simulink model "cmult_core"  (R2013a)
settings: Solver=ode45  StartTime=0.0  StopTime=10.0  RelTol=1e-3
libraries: xbsIndex_r4 x2035, casper_library_misc x116, casper_library_multipliers x36
(part 8 of 23)

== system cmult_core/vaccs/cplx_vacc13 ==
  new_acc : Inport
  din : Inport  Port=2
  c_to_ri : casper_library_misc/c_to_ri  n_bits=17  bin_pt=0
      settings: AttributesFormatString=17_0 r/i
  ri_to_c : casper_library_misc/ri_to_c
  simple_bram_vacc36 : Subsystem  AncestorBlock=casper_library_accumulators/simple_bram_vacc  mask(simple_bram_vacc){vec_len=vacc_len, arith_type=Signed, n_bits=32, bin_pt=0}
      mask prompts: vec_len "Vector length:"; arith_type "Output type:"; n_bits "Bit width (output):"; bin_pt "Binary point (output):"
      mask help: This simple vector accumulator is based on a shift register. It outputs its previous accumulated vector after a new_acc pulse is received.
      mask init:
      | simple_bram_vacc_init(gcb, ...
      |     'vec_len', vec_len, ...
      |     'arith_type', arith_type, ...
      |     'n_bits', n_bits, ...
      |     'bin_pt', bin_pt);
      mask TypeOptions arith_type: Signed | Unsigned
  simple_bram_vacc37 : Subsystem  AncestorBlock=casper_library_accumulators/simple_bram_vacc  mask(simple_bram_vacc){vec_len=vacc_len, arith_type=Signed, n_bits=32, bin_pt=0}
      mask prompts: vec_len "Vector length:"; arith_type "Output type:"; n_bits "Bit width (output):"; bin_pt "Binary point (output):"
      mask help: This simple vector accumulator is based on a shift register. It outputs its previous accumulated vector after a new_acc pulse is received.
      mask init:
      | simple_bram_vacc_init(gcb, ...
      |     'vec_len', vec_len, ...
      |     'arith_type', arith_type, ...
      |     'n_bits', n_bits, ...
      |     'bin_pt', bin_pt);
      mask TypeOptions arith_type: Signed | Unsigned
  dout : Outport
  vld : Outport  Port=2
  wires:
  din/1 -> c_to_ri/1
  simple_bram_vacc36/2(valid) -> vld/1
  simple_bram_vacc37/1(dout) -> ri_to_c/2
  simple_bram_vacc36/1(dout) -> ri_to_c/1
  c_to_ri/2 -> simple_bram_vacc37/2(din)
  new_acc/1 -> simple_bram_vacc36/1(new_acc), simple_bram_vacc37/1(new_acc)
  c_to_ri/1 -> simple_bram_vacc36/2(din)
  simple_bram_vacc37/2(valid) -> ?
  ri_to_c/1 -> dout/1

== system cmult_core/vaccs/cplx_vacc14 ==
  new_acc : Inport
  din : Inport  Port=2
  c_to_ri : casper_library_misc/c_to_ri  n_bits=17  bin_pt=0
      settings: AttributesFormatString=17_0 r/i
  ri_to_c : casper_library_misc/ri_to_c
  simple_bram_vacc36 : Subsystem  AncestorBlock=casper_library_accumulators/simple_bram_vacc  mask(simple_bram_vacc){vec_len=vacc_len, arith_type=Signed, n_bits=32, bin_pt=0}
      mask prompts: vec_len "Vector length:"; arith_type "Output type:"; n_bits "Bit width (output):"; bin_pt "Binary point (output):"
      mask help: This simple vector accumulator is based on a shift register. It outputs its previous accumulated vector after a new_acc pulse is received.
      mask init:
      | simple_bram_vacc_init(gcb, ...
      |     'vec_len', vec_len, ...
      |     'arith_type', arith_type, ...
      |     'n_bits', n_bits, ...
      |     'bin_pt', bin_pt);
      mask TypeOptions arith_type: Signed | Unsigned
  simple_bram_vacc37 : Subsystem  AncestorBlock=casper_library_accumulators/simple_bram_vacc  mask(simple_bram_vacc){vec_len=vacc_len, arith_type=Signed, n_bits=32, bin_pt=0}
      mask prompts: vec_len "Vector length:"; arith_type "Output type:"; n_bits "Bit width (output):"; bin_pt "Binary point (output):"
      mask help: This simple vector accumulator is based on a shift register. It outputs its previous accumulated vector after a new_acc pulse is received.
      mask init:
      | simple_bram_vacc_init(gcb, ...
      |     'vec_len', vec_len, ...
      |     'arith_type', arith_type, ...
      |     'n_bits', n_bits, ...
      |     'bin_pt', bin_pt);
      mask TypeOptions arith_type: Signed | Unsigned
  dout : Outport
  vld : Outport  Port=2
  wires:
  ri_to_c/1 -> dout/1
  simple_bram_vacc37/2(valid) -> ?
  c_to_ri/1 -> simple_bram_vacc36/2(din)
  new_acc/1 -> simple_bram_vacc37/1(new_acc), simple_bram_vacc36/1(new_acc)
  c_to_ri/2 -> simple_bram_vacc37/2(din)
  simple_bram_vacc36/1(dout) -> ri_to_c/1
  simple_bram_vacc37/1(dout) -> ri_to_c/2
  simple_bram_vacc36/2(valid) -> vld/1
  din/1 -> c_to_ri/1

== system cmult_core/vaccs/cplx_vacc15 ==
  new_acc : Inport
  din : Inport  Port=2
  c_to_ri : casper_library_misc/c_to_ri  n_bits=17  bin_pt=0
      settings: AttributesFormatString=17_0 r/i
  ri_to_c : casper_library_misc/ri_to_c
  simple_bram_vacc36 : Subsystem  AncestorBlock=casper_library_accumulators/simple_bram_vacc  mask(simple_bram_vacc){vec_len=vacc_len, arith_type=Signed, n_bits=32, bin_pt=0}
      mask prompts: vec_len "Vector length:"; arith_type "Output type:"; n_bits "Bit width (output):"; bin_pt "Binary point (output):"
      mask help: This simple vector accumulator is based on a shift register. It outputs its previous accumulated vector after a new_acc pulse is received.
      mask init:
      | simple_bram_vacc_init(gcb, ...
      |     'vec_len', vec_len, ...
      |     'arith_type', arith_type, ...
      |     'n_bits', n_bits, ...
      |     'bin_pt', bin_pt);
      mask TypeOptions arith_type: Signed | Unsigned
  simple_bram_vacc37 : Subsystem  AncestorBlock=casper_library_accumulators/simple_bram_vacc  mask(simple_bram_vacc){vec_len=vacc_len, arith_type=Signed, n_bits=32, bin_pt=0}
      mask prompts: vec_len "Vector length:"; arith_type "Output type:"; n_bits "Bit width (output):"; bin_pt "Binary point (output):"
      mask help: This simple vector accumulator is based on a shift register. It outputs its previous accumulated vector after a new_acc pulse is received.
      mask init:
      | simple_bram_vacc_init(gcb, ...
      |     'vec_len', vec_len, ...
      |     'arith_type', arith_type, ...
      |     'n_bits', n_bits, ...
      |     'bin_pt', bin_pt);
      mask TypeOptions arith_type: Signed | Unsigned
  dout : Outport
  vld : Outport  Port=2
  wires:
  din/1 -> c_to_ri/1
  simple_bram_vacc36/2(valid) -> vld/1
  simple_bram_vacc37/1(dout) -> ri_to_c/2
  simple_bram_vacc36/1(dout) -> ri_to_c/1
  c_to_ri/2 -> simple_bram_vacc37/2(din)
  new_acc/1 -> simple_bram_vacc36/1(new_acc), simple_bram_vacc37/1(new_acc)
  c_to_ri/1 -> simple_bram_vacc36/2(din)
  simple_bram_vacc37/2(valid) -> ?
  ri_to_c/1 -> dout/1

== system cmult_core/vaccs/cplx_vacc16 ==
  new_acc : Inport
  din : Inport  Port=2
  c_to_ri : casper_library_misc/c_to_ri  n_bits=17  bin_pt=0
      settings: AttributesFormatString=17_0 r/i
  ri_to_c : casper_library_misc/ri_to_c
  simple_bram_vacc36 : Subsystem  AncestorBlock=casper_library_accumulators/simple_bram_vacc  mask(simple_bram_vacc){vec_len=vacc_len, arith_type=Signed, n_bits=32, bin_pt=0}
      mask prompts: vec_len "Vector length:"; arith_type "Output type:"; n_bits "Bit width (output):"; bin_pt "Binary point (output):"
      mask help: This simple vector accumulator is based on a shift register. It outputs its previous accumulated vector after a new_acc pulse is received.
      mask init:
      | simple_bram_vacc_init(gcb, ...
      |     'vec_len', vec_len, ...
      |     'arith_type', arith_type, ...
      |     'n_bits', n_bits, ...
      |     'bin_pt', bin_pt);
      mask TypeOptions arith_type: Signed | Unsigned
  simple_bram_vacc37 : Subsystem  AncestorBlock=casper_library_accumulators/simple_bram_vacc  mask(simple_bram_vacc){vec_len=vacc_len, arith_type=Signed, n_bits=32, bin_pt=0}
      mask prompts: vec_len "Vector length:"; arith_type "Output type:"; n_bits "Bit width (output):"; bin_pt "Binary point (output):"
      mask help: This simple vector accumulator is based on a shift register. It outputs its previous accumulated vector after a new_acc pulse is received.
      mask init:
      | simple_bram_vacc_init(gcb, ...
      |     'vec_len', vec_len, ...
      |     'arith_type', arith_type, ...
      |     'n_bits', n_bits, ...
      |     'bin_pt', bin_pt);
      mask TypeOptions arith_type: Signed | Unsigned
  dout : Outport
  vld : Outport  Port=2
  wires:
  din/1 -> c_to_ri/1
  simple_bram_vacc36/2(valid) -> vld/1
  simple_bram_vacc37/1(dout) -> ri_to_c/2
  simple_bram_vacc36/1(dout) -> ri_to_c/1
  c_to_ri/2 -> simple_bram_vacc37/2(din)
  new_acc/1 -> simple_bram_vacc36/1(new_acc), simple_bram_vacc37/1(new_acc)
  c_to_ri/1 -> simple_bram_vacc36/2(din)
  simple_bram_vacc37/2(valid) -> ?
  ri_to_c/1 -> dout/1

== system cmult_core/vaccs/cplx_vacc17 ==
  new_acc : Inport
  din : Inport  Port=2
  c_to_ri : casper_library_misc/c_to_ri  n_bits=17  bin_pt=0
      settings: AttributesFormatString=17_0 r/i
  ri_to_c : casper_library_misc/ri_to_c
  simple_bram_vacc36 : Subsystem  AncestorBlock=casper_library_accumulators/simple_bram_vacc  mask(simple_bram_vacc){vec_len=vacc_len, arith_type=Signed, n_bits=32, bin_pt=0}
      mask prompts: vec_len "Vector length:"; arith_type "Output type:"; n_bits "Bit width (output):"; bin_pt "Binary point (output):"
      mask help: This simple vector accumulator is based on a shift register. It outputs its previous accumulated vector after a new_acc pulse is received.
      mask init:
      | simple_bram_vacc_init(gcb, ...
      |     'vec_len', vec_len, ...
      |     'arith_type', arith_type, ...
      |     'n_bits', n_bits, ...
      |     'bin_pt', bin_pt);
      mask TypeOptions arith_type: Signed | Unsigned
  simple_bram_vacc37 : Subsystem  AncestorBlock=casper_library_accumulators/simple_bram_vacc  mask(simple_bram_vacc){vec_len=vacc_len, arith_type=Signed, n_bits=32, bin_pt=0}
      mask prompts: vec_len "Vector length:"; arith_type "Output type:"; n_bits "Bit width (output):"; bin_pt "Binary point (output):"
      mask help: This simple vector accumulator is based on a shift register. It outputs its previous accumulated vector after a new_acc pulse is received.
      mask init:
      | simple_bram_vacc_init(gcb, ...
      |     'vec_len', vec_len, ...
      |     'arith_type', arith_type, ...
      |     'n_bits', n_bits, ...
      |     'bin_pt', bin_pt);
      mask TypeOptions arith_type: Signed | Unsigned
  dout : Outport
  vld : Outport  Port=2
  wires:
  ri_to_c/1 -> dout/1
  simple_bram_vacc37/2(valid) -> ?
  c_to_ri/1 -> simple_bram_vacc36/2(din)
  new_acc/1 -> simple_bram_vacc37/1(new_acc), simple_bram_vacc36/1(new_acc)
  c_to_ri/2 -> simple_bram_vacc37/2(din)
  simple_bram_vacc36/1(dout) -> ri_to_c/1
  simple_bram_vacc37/1(dout) -> ri_to_c/2
  simple_bram_vacc36/2(valid) -> vld/1
  din/1 -> c_to_ri/1

== system cmult_core/vaccs/cplx_vacc18 ==
  new_acc : Inport
  din : Inport  Port=2
  c_to_ri : casper_library_misc/c_to_ri  n_bits=17  bin_pt=0
      settings: AttributesFormatString=17_0 r/i
  ri_to_c : casper_library_misc/ri_to_c
  simple_bram_vacc36 : Subsystem  AncestorBlock=casper_library_accumulators/simple_bram_vacc  mask(simple_bram_vacc){vec_len=vacc_len, arith_type=Signed, n_bits=32, bin_pt=0}
      mask prompts: vec_len "Vector length:"; arith_type "Output type:"; n_bits "Bit width (output):"; bin_pt "Binary point (output):"
      mask help: This simple vector accumulator is based on a shift register. It outputs its previous accumulated vector after a new_acc pulse is received.
      mask init:
      | simple_bram_vacc_init(gcb, ...
      |     'vec_len', vec_len, ...
      |     'arith_type', arith_type, ...
      |     'n_bits', n_bits, ...
      |     'bin_pt', bin_pt);
      mask TypeOptions arith_type: Signed | Unsigned
  simple_bram_vacc37 : Subsystem  AncestorBlock=casper_library_accumulators/simple_bram_vacc  mask(simple_bram_vacc){vec_len=vacc_len, arith_type=Signed, n_bits=32, bin_pt=0}
      mask prompts: vec_len "Vector length:"; arith_type "Output type:"; n_bits "Bit width (output):"; bin_pt "Binary point (output):"
      mask help: This simple vector accumulator is based on a shift register. It outputs its previous accumulated vector after a new_acc pulse is received.
      mask init:
      | simple_bram_vacc_init(gcb, ...
      |     'vec_len', vec_len, ...
      |     'arith_type', arith_type, ...
      |     'n_bits', n_bits, ...
      |     'bin_pt', bin_pt);
      mask TypeOptions arith_type: Signed | Unsigned
  dout : Outport
  vld : Outport  Port=2
  wires:
  din/1 -> c_to_ri/1
  simple_bram_vacc36/2(valid) -> vld/1
  simple_bram_vacc37/1(dout) -> ri_to_c/2
  simple_bram_vacc36/1(dout) -> ri_to_c/1
  c_to_ri/2 -> simple_bram_vacc37/2(din)
  new_acc/1 -> simple_bram_vacc36/1(new_acc), simple_bram_vacc37/1(new_acc)
  c_to_ri/1 -> simple_bram_vacc36/2(din)
  simple_bram_vacc37/2(valid) -> ?
  ri_to_c/1 -> dout/1

== system cmult_core/vaccs/cplx_vacc19 ==
  new_acc : Inport
  din : Inport  Port=2
  c_to_ri : casper_library_misc/c_to_ri  n_bits=17  bin_pt=0
      settings: AttributesFormatString=17_0 r/i
  ri_to_c : casper_library_misc/ri_to_c
  simple_bram_vacc36 : Subsystem  AncestorBlock=casper_library_accumulators/simple_bram_vacc  mask(simple_bram_vacc){vec_len=vacc_len, arith_type=Signed, n_bits=32, bin_pt=0}
      mask prompts: vec_len "Vector length:"; arith_type "Output type:"; n_bits "Bit width (output):"; bin_pt "Binary point (output):"
      mask help: This simple vector accumulator is based on a shift register. It outputs its previous accumulated vector after a new_acc pulse is received.
      mask init:
      | simple_bram_vacc_init(gcb, ...
      |     'vec_len', vec_len, ...
      |     'arith_type', arith_type, ...
      |     'n_bits', n_bits, ...
      |     'bin_pt', bin_pt);
      mask TypeOptions arith_type: Signed | Unsigned
  simple_bram_vacc37 : Subsystem  AncestorBlock=casper_library_accumulators/simple_bram_vacc  mask(simple_bram_vacc){vec_len=vacc_len, arith_type=Signed, n_bits=32, bin_pt=0}
      mask prompts: vec_len "Vector length:"; arith_type "Output type:"; n_bits "Bit width (output):"; bin_pt "Binary point (output):"
      mask help: This simple vector accumulator is based on a shift register. It outputs its previous accumulated vector after a new_acc pulse is received.
      mask init:
      | simple_bram_vacc_init(gcb, ...
      |     'vec_len', vec_len, ...
      |     'arith_type', arith_type, ...
      |     'n_bits', n_bits, ...
      |     'bin_pt', bin_pt);
      mask TypeOptions arith_type: Signed | Unsigned
  dout : Outport
  vld : Outport  Port=2
  wires:
  ri_to_c/1 -> dout/1
  simple_bram_vacc37/2(valid) -> ?
  c_to_ri/1 -> simple_bram_vacc36/2(din)
  new_acc/1 -> simple_bram_vacc37/1(new_acc), simple_bram_vacc36/1(new_acc)
  c_to_ri/2 -> simple_bram_vacc37/2(din)
  simple_bram_vacc36/1(dout) -> ri_to_c/1
  simple_bram_vacc37/1(dout) -> ri_to_c/2
  simple_bram_vacc36/2(valid) -> vld/1
  din/1 -> c_to_ri/1

== system cmult_core/vaccs/cplx_vacc2 ==
  new_acc : Inport
  din : Inport  Port=2
  c_to_ri : casper_library_misc/c_to_ri  n_bits=17  bin_pt=0
      settings: AttributesFormatString=17_0 r/i
  ri_to_c : casper_library_misc/ri_to_c
  simple_bram_vacc36 : Subsystem  AncestorBlock=casper_library_accumulators/simple_bram_vacc  mask(simple_bram_vacc){vec_len=vacc_len, arith_type=Signed, n_bits=32, bin_pt=0}
      mask prompts: vec_len "Vector length:"; arith_type "Output type:"; n_bits "Bit width (output):"; bin_pt "Binary point (output):"
      mask help: This simple vector accumulator is based on a shift register. It outputs its previous accumulated vector after a new_acc pulse is received.
      mask init:
      | simple_bram_vacc_init(gcb, ...
      |     'vec_len', vec_len, ...
      |     'arith_type', arith_type, ...
      |     'n_bits', n_bits, ...
      |     'bin_pt', bin_pt);
      mask TypeOptions arith_type: Signed | Unsigned
  simple_bram_vacc37 : Subsystem  AncestorBlock=casper_library_accumulators/simple_bram_vacc  mask(simple_bram_vacc){vec_len=vacc_len, arith_type=Signed, n_bits=32, bin_pt=0}
      mask prompts: vec_len "Vector length:"; arith_type "Output type:"; n_bits "Bit width (output):"; bin_pt "Binary point (output):"
      mask help: This simple vector accumulator is based on a shift register. It outputs its previous accumulated vector after a new_acc pulse is received.
      mask init:
      | simple_bram_vacc_init(gcb, ...
      |     'vec_len', vec_len, ...
      |     'arith_type', arith_type, ...
      |     'n_bits', n_bits, ...
      |     'bin_pt', bin_pt);
      mask TypeOptions arith_type: Signed | Unsigned
  dout : Outport
  vld : Outport  Port=2
  wires:
  din/1 -> c_to_ri/1
  simple_bram_vacc36/2(valid) -> vld/1
  simple_bram_vacc37/1(dout) -> ri_to_c/2
  simple_bram_vacc36/1(dout) -> ri_to_c/1
  c_to_ri/2 -> simple_bram_vacc37/2(din)
  new_acc/1 -> simple_bram_vacc36/1(new_acc), simple_bram_vacc37/1(new_acc)
  c_to_ri/1 -> simple_bram_vacc36/2(din)
  simple_bram_vacc37/2(valid) -> ?
  ri_to_c/1 -> dout/1

== system cmult_core/vaccs/cplx_vacc20 ==
  new_acc : Inport
  din : Inport  Port=2
  c_to_ri : casper_library_misc/c_to_ri  n_bits=17  bin_pt=0
      settings: AttributesFormatString=17_0 r/i
  ri_to_c : casper_library_misc/ri_to_c
  simple_bram_vacc36 : Subsystem  AncestorBlock=casper_library_accumulators/simple_bram_vacc  mask(simple_bram_vacc){vec_len=vacc_len, arith_type=Signed, n_bits=32, bin_pt=0}
      mask prompts: vec_len "Vector length:"; arith_type "Output type:"; n_bits "Bit width (output):"; bin_pt "Binary point (output):"
      mask help: This simple vector accumulator is based on a shift register. It outputs its previous accumulated vector after a new_acc pulse is received.
      mask init:
      | simple_bram_vacc_init(gcb, ...
      |     'vec_len', vec_len, ...
      |     'arith_type', arith_type, ...
      |     'n_bits', n_bits, ...
      |     'bin_pt', bin_pt);
      mask TypeOptions arith_type: Signed | Unsigned
  simple_bram_vacc37 : Subsystem  AncestorBlock=casper_library_accumulators/simple_bram_vacc  mask(simple_bram_vacc){vec_len=vacc_len, arith_type=Signed, n_bits=32, bin_pt=0}
      mask prompts: vec_len "Vector length:"; arith_type "Output type:"; n_bits "Bit width (output):"; bin_pt "Binary point (output):"
      mask help: This simple vector accumulator is based on a shift register. It outputs its previous accumulated vector after a new_acc pulse is received.
      mask init:
      | simple_bram_vacc_init(gcb, ...
      |     'vec_len', vec_len, ...
      |     'arith_type', arith_type, ...
      |     'n_bits', n_bits, ...
      |     'bin_pt', bin_pt);
      mask TypeOptions arith_type: Signed | Unsigned
  dout : Outport
  vld : Outport  Port=2
  wires:
  din/1 -> c_to_ri/1
  simple_bram_vacc36/2(valid) -> vld/1
  simple_bram_vacc37/1(dout) -> ri_to_c/2
  simple_bram_vacc36/1(dout) -> ri_to_c/1
  c_to_ri/2 -> simple_bram_vacc37/2(din)
  new_acc/1 -> simple_bram_vacc36/1(new_acc), simple_bram_vacc37/1(new_acc)
  c_to_ri/1 -> simple_bram_vacc36/2(din)
  simple_bram_vacc37/2(valid) -> ?
  ri_to_c/1 -> dout/1

== system cmult_core/vaccs/cplx_vacc21 ==
  new_acc : Inport
  din : Inport  Port=2
  c_to_ri : casper_library_misc/c_to_ri  n_bits=17  bin_pt=0
      settings: AttributesFormatString=17_0 r/i
  ri_to_c : casper_library_misc/ri_to_c
  simple_bram_vacc36 : Subsystem  AncestorBlock=casper_library_accumulators/simple_bram_vacc  mask(simple_bram_vacc){vec_len=vacc_len, arith_type=Signed, n_bits=32, bin_pt=0}
      mask prompts: vec_len "Vector length:"; arith_type "Output type:"; n_bits "Bit width (output):"; bin_pt "Binary point (output):"
      mask help: This simple vector accumulator is based on a shift register. It outputs its previous accumulated vector after a new_acc pulse is received.
      mask init:
      | simple_bram_vacc_init(gcb, ...
      |     'vec_len', vec_len, ...
      |     'arith_type', arith_type, ...
      |     'n_bits', n_bits, ...
      |     'bin_pt', bin_pt);
      mask TypeOptions arith_type: Signed | Unsigned
  simple_bram_vacc37 : Subsystem  AncestorBlock=casper_library_accumulators/simple_bram_vacc  mask(simple_bram_vacc){vec_len=vacc_len, arith_type=Signed, n_bits=32, bin_pt=0}
      mask prompts: vec_len "Vector length:"; arith_type "Output type:"; n_bits "Bit width (output):"; bin_pt "Binary point (output):"
      mask help: This simple vector accumulator is based on a shift register. It outputs its previous accumulated vector after a new_acc pulse is received.
      mask init:
      | simple_bram_vacc_init(gcb, ...
      |     'vec_len', vec_len, ...
      |     'arith_type', arith_type, ...
      |     'n_bits', n_bits, ...
      |     'bin_pt', bin_pt);
      mask TypeOptions arith_type: Signed | Unsigned
  dout : Outport
  vld : Outport  Port=2
  wires:
  ri_to_c/1 -> dout/1
  simple_bram_vacc37/2(valid) -> ?
  c_to_ri/1 -> simple_bram_vacc36/2(din)
  new_acc/1 -> simple_bram_vacc37/1(new_acc), simple_bram_vacc36/1(new_acc)
  c_to_ri/2 -> simple_bram_vacc37/2(din)
  simple_bram_vacc36/1(dout) -> ri_to_c/1
  simple_bram_vacc37/1(dout) -> ri_to_c/2
  simple_bram_vacc36/2(valid) -> vld/1
  din/1 -> c_to_ri/1

== system cmult_core/vaccs/cplx_vacc22 ==
  new_acc : Inport
  din : Inport  Port=2
  c_to_ri : casper_library_misc/c_to_ri  n_bits=17  bin_pt=0
      settings: AttributesFormatString=17_0 r/i
  ri_to_c : casper_library_misc/ri_to_c
  simple_bram_vacc36 : Subsystem  AncestorBlock=casper_library_accumulators/simple_bram_vacc  mask(simple_bram_vacc){vec_len=vacc_len, arith_type=Signed, n_bits=32, bin_pt=0}
      mask prompts: vec_len "Vector length:"; arith_type "Output type:"; n_bits "Bit width (output):"; bin_pt "Binary point (output):"
      mask help: This simple vector accumulator is based on a shift register. It outputs its previous accumulated vector after a new_acc pulse is received.
      mask init:
      | simple_bram_vacc_init(gcb, ...
      |     'vec_len', vec_len, ...
      |     'arith_type', arith_type, ...
      |     'n_bits', n_bits, ...
      |     'bin_pt', bin_pt);
      mask TypeOptions arith_type: Signed | Unsigned
  simple_bram_vacc37 : Subsystem  AncestorBlock=casper_library_accumulators/simple_bram_vacc  mask(simple_bram_vacc){vec_len=vacc_len, arith_type=Signed, n_bits=32, bin_pt=0}
      mask prompts: vec_len "Vector length:"; arith_type "Output type:"; n_bits "Bit width (output):"; bin_pt "Binary point (output):"
      mask help: This simple vector accumulator is based on a shift register. It outputs its previous accumulated vector after a new_acc pulse is received.
      mask init:
      | simple_bram_vacc_init(gcb, ...
      |     'vec_len', vec_len, ...
      |     'arith_type', arith_type, ...
      |     'n_bits', n_bits, ...
      |     'bin_pt', bin_pt);
      mask TypeOptions arith_type: Signed | Unsigned
  dout : Outport
  vld : Outport  Port=2
  wires:
  ri_to_c/1 -> dout/1
  simple_bram_vacc37/2(valid) -> ?
  c_to_ri/1 -> simple_bram_vacc36/2(din)
  new_acc/1 -> simple_bram_vacc37/1(new_acc), simple_bram_vacc36/1(new_acc)
  c_to_ri/2 -> simple_bram_vacc37/2(din)
  simple_bram_vacc36/1(dout) -> ri_to_c/1
  simple_bram_vacc37/1(dout) -> ri_to_c/2
  simple_bram_vacc36/2(valid) -> vld/1
  din/1 -> c_to_ri/1

== system cmult_core/vaccs/cplx_vacc23 ==
  new_acc : Inport
  din : Inport  Port=2
  c_to_ri : casper_library_misc/c_to_ri  n_bits=17  bin_pt=0
      settings: AttributesFormatString=17_0 r/i
  ri_to_c : casper_library_misc/ri_to_c
  simple_bram_vacc36 : Subsystem  AncestorBlock=casper_library_accumulators/simple_bram_vacc  mask(simple_bram_vacc){vec_len=vacc_len, arith_type=Signed, n_bits=32, bin_pt=0}
      mask prompts: vec_len "Vector length:"; arith_type "Output type:"; n_bits "Bit width (output):"; bin_pt "Binary point (output):"
      mask help: This simple vector accumulator is based on a shift register. It outputs its previous accumulated vector after a new_acc pulse is received.
      mask init:
      | simple_bram_vacc_init(gcb, ...
      |     'vec_len', vec_len, ...
      |     'arith_type', arith_type, ...
      |     'n_bits', n_bits, ...
      |     'bin_pt', bin_pt);
      mask TypeOptions arith_type: Signed | Unsigned
  simple_bram_vacc37 : Subsystem  AncestorBlock=casper_library_accumulators/simple_bram_vacc  mask(simple_bram_vacc){vec_len=vacc_len, arith_type=Signed, n_bits=32, bin_pt=0}
      mask prompts: vec_len "Vector length:"; arith_type "Output type:"; n_bits "Bit width (output):"; bin_pt "Binary point (output):"
      mask help: This simple vector accumulator is based on a shift register. It outputs its previous accumulated vector after a new_acc pulse is received.
      mask init:
      | simple_bram_vacc_init(gcb, ...
      |     'vec_len', vec_len, ...
      |     'arith_type', arith_type, ...
      |     'n_bits', n_bits, ...
      |     'bin_pt', bin_pt);
      mask TypeOptions arith_type: Signed | Unsigned
  dout : Outport
  vld : Outport  Port=2
  wires:
  din/1 -> c_to_ri/1
  simple_bram_vacc36/2(valid) -> vld/1
  simple_bram_vacc37/1(dout) -> ri_to_c/2
  simple_bram_vacc36/1(dout) -> ri_to_c/1
  c_to_ri/2 -> simple_bram_vacc37/2(din)
  new_acc/1 -> simple_bram_vacc36/1(new_acc), simple_bram_vacc37/1(new_acc)
  c_to_ri/1 -> simple_bram_vacc36/2(din)
  simple_bram_vacc37/2(valid) -> ?
  ri_to_c/1 -> dout/1

== system cmult_core/vaccs/cplx_vacc24 ==
  new_acc : Inport
  din : Inport  Port=2
  c_to_ri : casper_library_misc/c_to_ri  n_bits=17  bin_pt=0
      settings: AttributesFormatString=17_0 r/i
  ri_to_c : casper_library_misc/ri_to_c
  simple_bram_vacc36 : Subsystem  AncestorBlock=casper_library_accumulators/simple_bram_vacc  mask(simple_bram_vacc){vec_len=vacc_len, arith_type=Signed, n_bits=32, bin_pt=0}
      mask prompts: vec_len "Vector length:"; arith_type "Output type:"; n_bits "Bit width (output):"; bin_pt "Binary point (output):"
      mask help: This simple vector accumulator is based on a shift register. It outputs its previous accumulated vector after a new_acc pulse is received.
      mask init:
      | simple_bram_vacc_init(gcb, ...
      |     'vec_len', vec_len, ...
      |     'arith_type', arith_type, ...
      |     'n_bits', n_bits, ...
      |     'bin_pt', bin_pt);
      mask TypeOptions arith_type: Signed | Unsigned
  simple_bram_vacc37 : Subsystem  AncestorBlock=casper_library_accumulators/simple_bram_vacc  mask(simple_bram_vacc){vec_len=vacc_len, arith_type=Signed, n_bits=32, bin_pt=0}
      mask prompts: vec_len "Vector length:"; arith_type "Output type:"; n_bits "Bit width (output):"; bin_pt "Binary point (output):"
      mask help: This simple vector accumulator is based on a shift register. It outputs its previous accumulated vector after a new_acc pulse is received.
      mask init:
      | simple_bram_vacc_init(gcb, ...
      |     'vec_len', vec_len, ...
      |     'arith_type', arith_type, ...
      |     'n_bits', n_bits, ...
      |     'bin_pt', bin_pt);
      mask TypeOptions arith_type: Signed | Unsigned
  dout : Outport
  vld : Outport  Port=2
  wires:
  din/1 -> c_to_ri/1
  simple_bram_vacc36/2(valid) -> vld/1
  simple_bram_vacc37/1(dout) -> ri_to_c/2
  simple_bram_vacc36/1(dout) -> ri_to_c/1
  c_to_ri/2 -> simple_bram_vacc37/2(din)
  new_acc/1 -> simple_bram_vacc36/1(new_acc), simple_bram_vacc37/1(new_acc)
  c_to_ri/1 -> simple_bram_vacc36/2(din)
  simple_bram_vacc37/2(valid) -> ?
  ri_to_c/1 -> dout/1

== system cmult_core/vaccs/cplx_vacc25 ==
  new_acc : Inport
  din : Inport  Port=2
  c_to_ri : casper_library_misc/c_to_ri  n_bits=17  bin_pt=0
      settings: AttributesFormatString=17_0 r/i
  ri_to_c : casper_library_misc/ri_to_c
  simple_bram_vacc36 : Subsystem  AncestorBlock=casper_library_accumulators/simple_bram_vacc  mask(simple_bram_vacc){vec_len=vacc_len, arith_type=Signed, n_bits=32, bin_pt=0}
      mask prompts: vec_len "Vector length:"; arith_type "Output type:"; n_bits "Bit width (output):"; bin_pt "Binary point (output):"
      mask help: This simple vector accumulator is based on a shift register. It outputs its previous accumulated vector after a new_acc pulse is received.
      mask init:
      | simple_bram_vacc_init(gcb, ...
      |     'vec_len', vec_len, ...
      |     'arith_type', arith_type, ...
      |     'n_bits', n_bits, ...
      |     'bin_pt', bin_pt);
      mask TypeOptions arith_type: Signed | Unsigned
  simple_bram_vacc37 : Subsystem  AncestorBlock=casper_library_accumulators/simple_bram_vacc  mask(simple_bram_vacc){vec_len=vacc_len, arith_type=Signed, n_bits=32, bin_pt=0}
      mask prompts: vec_len "Vector length:"; arith_type "Output type:"; n_bits "Bit width (output):"; bin_pt "Binary point (output):"
      mask help: This simple vector accumulator is based on a shift register. It outputs its previous accumulated vector after a new_acc pulse is received.
      mask init:
      | simple_bram_vacc_init(gcb, ...
      |     'vec_len', vec_len, ...
      |     'arith_type', arith_type, ...
      |     'n_bits', n_bits, ...
      |     'bin_pt', bin_pt);
      mask TypeOptions arith_type: Signed | Unsigned
  dout : Outport
  vld : Outport  Port=2
  wires:
  ri_to_c/1 -> dout/1
  simple_bram_vacc37/2(valid) -> ?
  c_to_ri/1 -> simple_bram_vacc36/2(din)
  new_acc/1 -> simple_bram_vacc37/1(new_acc), simple_bram_vacc36/1(new_acc)
  c_to_ri/2 -> simple_bram_vacc37/2(din)
  simple_bram_vacc36/1(dout) -> ri_to_c/1
  simple_bram_vacc37/1(dout) -> ri_to_c/2
  simple_bram_vacc36/2(valid) -> vld/1
  din/1 -> c_to_ri/1

== system cmult_core/vaccs/cplx_vacc26 ==
  new_acc : Inport
  din : Inport  Port=2
  c_to_ri : casper_library_misc/c_to_ri  n_bits=17  bin_pt=0
      settings: AttributesFormatString=17_0 r/i
  ri_to_c : casper_library_misc/ri_to_c
  simple_bram_vacc36 : Subsystem  AncestorBlock=casper_library_accumulators/simple_bram_vacc  mask(simple_bram_vacc){vec_len=vacc_len, arith_type=Signed, n_bits=32, bin_pt=0}
      mask prompts: vec_len "Vector length:"; arith_type "Output type:"; n_bits "Bit width (output):"; bin_pt "Binary point (output):"
      mask help: This simple vector accumulator is based on a shift register. It outputs its previous accumulated vector after a new_acc pulse is received.
      mask init:
      | simple_bram_vacc_init(gcb, ...
      |     'vec_len', vec_len, ...
      |     'arith_type', arith_type, ...
      |     'n_bits', n_bits, ...
      |     'bin_pt', bin_pt);
      mask TypeOptions arith_type: Signed | Unsigned
  simple_bram_vacc37 : Subsystem  AncestorBlock=casper_library_accumulators/simple_bram_vacc  mask(simple_bram_vacc){vec_len=vacc_len, arith_type=Signed, n_bits=32, bin_pt=0}
      mask prompts: vec_len "Vector length:"; arith_type "Output type:"; n_bits "Bit width (output):"; bin_pt "Binary point (output):"
      mask help: This simple vector accumulator is based on a shift register. It outputs its previous accumulated vector after a new_acc pulse is received.
      mask init:
      | simple_bram_vacc_init(gcb, ...
      |     'vec_len', vec_len, ...
      |     'arith_type', arith_type, ...
      |     'n_bits', n_bits, ...
      |     'bin_pt', bin_pt);
      mask TypeOptions arith_type: Signed | Unsigned
  dout : Outport
  vld : Outport  Port=2
  wires:
  din/1 -> c_to_ri/1
  simple_bram_vacc36/2(valid) -> vld/1
  simple_bram_vacc37/1(dout) -> ri_to_c/2
  simple_bram_vacc36/1(dout) -> ri_to_c/1
  c_to_ri/2 -> simple_bram_vacc37/2(din)
  new_acc/1 -> simple_bram_vacc36/1(new_acc), simple_bram_vacc37/1(new_acc)
  c_to_ri/1 -> simple_bram_vacc36/2(din)
  simple_bram_vacc37/2(valid) -> ?
  ri_to_c/1 -> dout/1

== system cmult_core/vaccs/cplx_vacc27 ==
  new_acc : Inport
  din : Inport  Port=2
  c_to_ri : casper_library_misc/c_to_ri  n_bits=17  bin_pt=0
      settings: AttributesFormatString=17_0 r/i
  ri_to_c : casper_library_misc/ri_to_c
  simple_bram_vacc36 : Subsystem  AncestorBlock=casper_library_accumulators/simple_bram_vacc  mask(simple_bram_vacc){vec_len=vacc_len, arith_type=Signed, n_bits=32, bin_pt=0}
      mask prompts: vec_len "Vector length:"; arith_type "Output type:"; n_bits "Bit width (output):"; bin_pt "Binary point (output):"
      mask help: This simple vector accumulator is based on a shift register. It outputs its previous accumulated vector after a new_acc pulse is received.
      mask init:
      | simple_bram_vacc_init(gcb, ...
      |     'vec_len', vec_len, ...
      |     'arith_type', arith_type, ...
      |     'n_bits', n_bits, ...
      |     'bin_pt', bin_pt);
      mask TypeOptions arith_type: Signed | Unsigned
  simple_bram_vacc37 : Subsystem  AncestorBlock=casper_library_accumulators/simple_bram_vacc  mask(simple_bram_vacc){vec_len=vacc_len, arith_type=Signed, n_bits=32, bin_pt=0}
      mask prompts: vec_len "Vector length:"; arith_type "Output type:"; n_bits "Bit width (output):"; bin_pt "Binary point (output):"
      mask help: This simple vector accumulator is based on a shift register. It outputs its previous accumulated vector after a new_acc pulse is received.
      mask init:
      | simple_bram_vacc_init(gcb, ...
      |     'vec_len', vec_len, ...
      |     'arith_type', arith_type, ...
      |     'n_bits', n_bits, ...
      |     'bin_pt', bin_pt);
      mask TypeOptions arith_type: Signed | Unsigned
  dout : Outport
  vld : Outport  Port=2
  wires:
  ri_to_c/1 -> dout/1
  simple_bram_vacc37/2(valid) -> ?
  c_to_ri/1 -> simple_bram_vacc36/2(din)
  new_acc/1 -> simple_bram_vacc37/1(new_acc), simple_bram_vacc36/1(new_acc)
  c_to_ri/2 -> simple_bram_vacc37/2(din)
  simple_bram_vacc36/1(dout) -> ri_to_c/1
  simple_bram_vacc37/1(dout) -> ri_to_c/2
  simple_bram_vacc36/2(valid) -> vld/1
  din/1 -> c_to_ri/1

== system cmult_core/vaccs/cplx_vacc28 ==
  new_acc : Inport
  din : Inport  Port=2
  c_to_ri : casper_library_misc/c_to_ri  n_bits=17  bin_pt=0
      settings: AttributesFormatString=17_0 r/i
  ri_to_c : casper_library_misc/ri_to_c
  simple_bram_vacc36 : Subsystem  AncestorBlock=casper_library_accumulators/simple_bram_vacc  mask(simple_bram_vacc){vec_len=vacc_len, arith_type=Signed, n_bits=32, bin_pt=0}
      mask prompts: vec_len "Vector length:"; arith_type "Output type:"; n_bits "Bit width (output):"; bin_pt "Binary point (output):"
      mask help: This simple vector accumulator is based on a shift register. It outputs its previous accumulated vector after a new_acc pulse is received.
      mask init:
      | simple_bram_vacc_init(gcb, ...
      |     'vec_len', vec_len, ...
      |     'arith_type', arith_type, ...
      |     'n_bits', n_bits, ...
      |     'bin_pt', bin_pt);
      mask TypeOptions arith_type: Signed | Unsigned
  simple_bram_vacc37 : Subsystem  AncestorBlock=casper_library_accumulators/simple_bram_vacc  mask(simple_bram_vacc){vec_len=vacc_len, arith_type=Signed, n_bits=32, bin_pt=0}
      mask prompts: vec_len "Vector length:"; arith_type "Output type:"; n_bits "Bit width (output):"; bin_pt "Binary point (output):"
      mask help: This simple vector accumulator is based on a shift register. It outputs its previous accumulated vector after a new_acc pulse is received.
      mask init:
      | simple_bram_vacc_init(gcb, ...
      |     'vec_len', vec_len, ...
      |     'arith_type', arith_type, ...
      |     'n_bits', n_bits, ...
      |     'bin_pt', bin_pt);
      mask TypeOptions arith_type: Signed | Unsigned
  dout : Outport
  vld : Outport  Port=2
  wires:
  ri_to_c/1 -> dout/1
  simple_bram_vacc37/2(valid) -> ?
  c_to_ri/1 -> simple_bram_vacc36/2(din)
  new_acc/1 -> simple_bram_vacc37/1(new_acc), simple_bram_vacc36/1(new_acc)
  c_to_ri/2 -> simple_bram_vacc37/2(din)
  simple_bram_vacc36/1(dout) -> ri_to_c/1
  simple_bram_vacc37/1(dout) -> ri_to_c/2
  simple_bram_vacc36/2(valid) -> vld/1
  din/1 -> c_to_ri/1

== system cmult_core/vaccs/cplx_vacc29 ==
  new_acc : Inport
  din : Inport  Port=2
  c_to_ri : casper_library_misc/c_to_ri  n_bits=17  bin_pt=0
      settings: AttributesFormatString=17_0 r/i
  ri_to_c : casper_library_misc/ri_to_c
  simple_bram_vacc36 : Subsystem  AncestorBlock=casper_library_accumulators/simple_bram_vacc  mask(simple_bram_vacc){vec_len=vacc_len, arith_type=Signed, n_bits=32, bin_pt=0}
      mask prompts: vec_len "Vector length:"; arith_type "Output type:"; n_bits "Bit width (output):"; bin_pt "Binary point (output):"
      mask help: This simple vector accumulator is based on a shift register. It outputs its previous accumulated vector after a new_acc pulse is received.
      mask init:
      | simple_bram_vacc_init(gcb, ...
      |     'vec_len', vec_len, ...
      |     'arith_type', arith_type, ...
      |     'n_bits', n_bits, ...
      |     'bin_pt', bin_pt);
      mask TypeOptions arith_type: Signed | Unsigned
  simple_bram_vacc37 : Subsystem  AncestorBlock=casper_library_accumulators/simple_bram_vacc  mask(simple_bram_vacc){vec_len=vacc_len, arith_type=Signed, n_bits=32, bin_pt=0}
      mask prompts: vec_len "Vector length:"; arith_type "Output type:"; n_bits "Bit width (output):"; bin_pt "Binary point (output):"
      mask help: This simple vector accumulator is based on a shift register. It outputs its previous accumulated vector after a new_acc pulse is received.
      mask init:
      | simple_bram_vacc_init(gcb, ...
      |     'vec_len', vec_len, ...
      |     'arith_type', arith_type, ...
      |     'n_bits', n_bits, ...
      |     'bin_pt', bin_pt);
      mask TypeOptions arith_type: Signed | Unsigned
  dout : Outport
  vld : Outport  Port=2
  wires:
  din/1 -> c_to_ri/1
  simple_bram_vacc36/2(valid) -> vld/1
  simple_bram_vacc37/1(dout) -> ri_to_c/2
  simple_bram_vacc36/1(dout) -> ri_to_c/1
  c_to_ri/2 -> simple_bram_vacc37/2(din)
  new_acc/1 -> simple_bram_vacc36/1(new_acc), simple_bram_vacc37/1(new_acc)
  c_to_ri/1 -> simple_bram_vacc36/2(din)
  simple_bram_vacc37/2(valid) -> ?
  ri_to_c/1 -> dout/1

== system cmult_core/vaccs/cplx_vacc3 ==
  new_acc : Inport
  din : Inport  Port=2
  c_to_ri : casper_library_misc/c_to_ri  n_bits=17  bin_pt=0
      settings: AttributesFormatString=17_0 r/i
  ri_to_c : casper_library_misc/ri_to_c
  simple_bram_vacc36 : Subsystem  AncestorBlock=casper_library_accumulators/simple_bram_vacc  mask(simple_bram_vacc){vec_len=vacc_len, arith_type=Signed, n_bits=32, bin_pt=0}
      mask prompts: vec_len "Vector length:"; arith_type "Output type:"; n_bits "Bit width (output):"; bin_pt "Binary point (output):"
      mask help: This simple vector accumulator is based on a shift register. It outputs its previous accumulated vector after a new_acc pulse is received.
      mask init:
      | simple_bram_vacc_init(gcb, ...
      |     'vec_len', vec_len, ...
      |     'arith_type', arith_type, ...
      |     'n_bits', n_bits, ...
      |     'bin_pt', bin_pt);
      mask TypeOptions arith_type: Signed | Unsigned
  simple_bram_vacc37 : Subsystem  AncestorBlock=casper_library_accumulators/simple_bram_vacc  mask(simple_bram_vacc){vec_len=vacc_len, arith_type=Signed, n_bits=32, bin_pt=0}
      mask prompts: vec_len "Vector length:"; arith_type "Output type:"; n_bits "Bit width (output):"; bin_pt "Binary point (output):"
      mask help: This simple vector accumulator is based on a shift register. It outputs its previous accumulated vector after a new_acc pulse is received.
      mask init:
      | simple_bram_vacc_init(gcb, ...
      |     'vec_len', vec_len, ...
      |     'arith_type', arith_type, ...
      |     'n_bits', n_bits, ...
      |     'bin_pt', bin_pt);
      mask TypeOptions arith_type: Signed | Unsigned
  dout : Outport
  vld : Outport  Port=2
  wires:
  ri_to_c/1 -> dout/1
  simple_bram_vacc37/2(valid) -> ?
  c_to_ri/1 -> simple_bram_vacc36/2(din)
  new_acc/1 -> simple_bram_vacc37/1(new_acc), simple_bram_vacc36/1(new_acc)
  c_to_ri/2 -> simple_bram_vacc37/2(din)
  simple_bram_vacc36/1(dout) -> ri_to_c/1
  simple_bram_vacc37/1(dout) -> ri_to_c/2
  simple_bram_vacc36/2(valid) -> vld/1
  din/1 -> c_to_ri/1

== system cmult_core/vaccs/cplx_vacc30 ==
  new_acc : Inport
  din : Inport  Port=2
  c_to_ri : casper_library_misc/c_to_ri  n_bits=17  bin_pt=0
      settings: AttributesFormatString=17_0 r/i
  ri_to_c : casper_library_misc/ri_to_c
  simple_bram_vacc36 : Subsystem  AncestorBlock=casper_library_accumulators/simple_bram_vacc  mask(simple_bram_vacc){vec_len=vacc_len, arith_type=Signed, n_bits=32, bin_pt=0}
      mask prompts: vec_len "Vector length:"; arith_type "Output type:"; n_bits "Bit width (output):"; bin_pt "Binary point (output):"
      mask help: This simple vector accumulator is based on a shift register. It outputs its previous accumulated vector after a new_acc pulse is received.
      mask init:
      | simple_bram_vacc_init(gcb, ...
      |     'vec_len', vec_len, ...
      |     'arith_type', arith_type, ...
      |     'n_bits', n_bits, ...
      |     'bin_pt', bin_pt);
      mask TypeOptions arith_type: Signed | Unsigned
  simple_bram_vacc37 : Subsystem  AncestorBlock=casper_library_accumulators/simple_bram_vacc  mask(simple_bram_vacc){vec_len=vacc_len, arith_type=Signed, n_bits=32, bin_pt=0}
      mask prompts: vec_len "Vector length:"; arith_type "Output type:"; n_bits "Bit width (output):"; bin_pt "Binary point (output):"
      mask help: This simple vector accumulator is based on a shift register. It outputs its previous accumulated vector after a new_acc pulse is received.
      mask init:
      | simple_bram_vacc_init(gcb, ...
      |     'vec_len', vec_len, ...
      |     'arith_type', arith_type, ...
      |     'n_bits', n_bits, ...
      |     'bin_pt', bin_pt);
      mask TypeOptions arith_type: Signed | Unsigned
  dout : Outport
  vld : Outport  Port=2
  wires:
  ri_to_c/1 -> dout/1
  simple_bram_vacc37/2(valid) -> ?
  c_to_ri/1 -> simple_bram_vacc36/2(din)
  new_acc/1 -> simple_bram_vacc37/1(new_acc), simple_bram_vacc36/1(new_acc)
  c_to_ri/2 -> simple_bram_vacc37/2(din)
  simple_bram_vacc36/1(dout) -> ri_to_c/1
  simple_bram_vacc37/1(dout) -> ri_to_c/2
  simple_bram_vacc36/2(valid) -> vld/1
  din/1 -> c_to_ri/1

== system cmult_core/vaccs/cplx_vacc31 ==
  new_acc : Inport
  din : Inport  Port=2
  c_to_ri : casper_library_misc/c_to_ri  n_bits=17  bin_pt=0
      settings: AttributesFormatString=17_0 r/i
  ri_to_c : casper_library_misc/ri_to_c
  simple_bram_vacc36 : Subsystem  AncestorBlock=casper_library_accumulators/simple_bram_vacc  mask(simple_bram_vacc){vec_len=vacc_len, arith_type=Signed, n_bits=32, bin_pt=0}
      mask prompts: vec_len "Vector length:"; arith_type "Output type:"; n_bits "Bit width (output):"; bin_pt "Binary point (output):"
      mask help: This simple vector accumulator is based on a shift register. It outputs its previous accumulated vector after a new_acc pulse is received.
      mask init:
      | simple_bram_vacc_init(gcb, ...
      |     'vec_len', vec_len, ...
      |     'arith_type', arith_type, ...
      |     'n_bits', n_bits, ...
      |     'bin_pt', bin_pt);
      mask TypeOptions arith_type: Signed | Unsigned
  simple_bram_vacc37 : Subsystem  AncestorBlock=casper_library_accumulators/simple_bram_vacc  mask(simple_bram_vacc){vec_len=vacc_len, arith_type=Signed, n_bits=32, bin_pt=0}
      mask prompts: vec_len "Vector length:"; arith_type "Output type:"; n_bits "Bit width (output):"; bin_pt "Binary point (output):"
      mask help: This simple vector accumulator is based on a shift register. It outputs its previous accumulated vector after a new_acc pulse is received.
      mask init:
      | simple_bram_vacc_init(gcb, ...
      |     'vec_len', vec_len, ...
      |     'arith_type', arith_type, ...
      |     'n_bits', n_bits, ...
      |     'bin_pt', bin_pt);
      mask TypeOptions arith_type: Signed | Unsigned
  dout : Outport
  vld : Outport  Port=2
  wires:
  din/1 -> c_to_ri/1
  simple_bram_vacc36/2(valid) -> vld/1
  simple_bram_vacc37/1(dout) -> ri_to_c/2
  simple_bram_vacc36/1(dout) -> ri_to_c/1
  c_to_ri/2 -> simple_bram_vacc37/2(din)
  new_acc/1 -> simple_bram_vacc36/1(new_acc), simple_bram_vacc37/1(new_acc)
  c_to_ri/1 -> simple_bram_vacc36/2(din)
  simple_bram_vacc37/2(valid) -> ?
  ri_to_c/1 -> dout/1

== system cmult_core/vaccs/cplx_vacc32 ==
  new_acc : Inport
  din : Inport  Port=2
  c_to_ri : casper_library_misc/c_to_ri  n_bits=17  bin_pt=0
      settings: AttributesFormatString=17_0 r/i
  ri_to_c : casper_library_misc/ri_to_c
  simple_bram_vacc36 : Subsystem  AncestorBlock=casper_library_accumulators/simple_bram_vacc  mask(simple_bram_vacc){vec_len=vacc_len, arith_type=Signed, n_bits=32, bin_pt=0}
      mask prompts: vec_len "Vector length:"; arith_type "Output type:"; n_bits "Bit width (output):"; bin_pt "Binary point (output):"
      mask help: This simple vector accumulator is based on a shift register. It outputs its previous accumulated vector after a new_acc pulse is received.
      mask init:
      | simple_bram_vacc_init(gcb, ...
      |     'vec_len', vec_len, ...
      |     'arith_type', arith_type, ...
      |     'n_bits', n_bits, ...
      |     'bin_pt', bin_pt);
      mask TypeOptions arith_type: Signed | Unsigned
  simple_bram_vacc37 : Subsystem  AncestorBlock=casper_library_accumulators/simple_bram_vacc  mask(simple_bram_vacc){vec_len=vacc_len, arith_type=Signed, n_bits=32, bin_pt=0}
      mask prompts: vec_len "Vector length:"; arith_type "Output type:"; n_bits "Bit width (output):"; bin_pt "Binary point (output):"
      mask help: This simple vector accumulator is based on a shift register. It outputs its previous accumulated vector after a new_acc pulse is received.
      mask init:
      | simple_bram_vacc_init(gcb, ...
      |     'vec_len', vec_len, ...
      |     'arith_type', arith_type, ...
      |     'n_bits', n_bits, ...
      |     'bin_pt', bin_pt);
      mask TypeOptions arith_type: Signed | Unsigned
  dout : Outport
  vld : Outport  Port=2
  wires:
  ri_to_c/1 -> dout/1
  simple_bram_vacc37/2(valid) -> ?
  c_to_ri/1 -> simple_bram_vacc36/2(din)
  new_acc/1 -> simple_bram_vacc37/1(new_acc), simple_bram_vacc36/1(new_acc)
  c_to_ri/2 -> simple_bram_vacc37/2(din)
  simple_bram_vacc36/1(dout) -> ri_to_c/1
  simple_bram_vacc37/1(dout) -> ri_to_c/2
  simple_bram_vacc36/2(valid) -> vld/1
  din/1 -> c_to_ri/1

== system cmult_core/vaccs/cplx_vacc33 ==
  new_acc : Inport
  din : Inport  Port=2
  c_to_ri : casper_library_misc/c_to_ri  n_bits=17  bin_pt=0
      settings: AttributesFormatString=17_0 r/i
  ri_to_c : casper_library_misc/ri_to_c
  simple_bram_vacc36 : Subsystem  AncestorBlock=casper_library_accumulators/simple_bram_vacc  mask(simple_bram_vacc){vec_len=vacc_len, arith_type=Signed, n_bits=32, bin_pt=0}
      mask prompts: vec_len "Vector length:"; arith_type "Output type:"; n_bits "Bit width (output):"; bin_pt "Binary point (output):"
      mask help: This simple vector accumulator is based on a shift register. It outputs its previous accumulated vector after a new_acc pulse is received.
      mask init:
      | simple_bram_vacc_init(gcb, ...
      |     'vec_len', vec_len, ...
      |     'arith_type', arith_type, ...
      |     'n_bits', n_bits, ...
      |     'bin_pt', bin_pt);
      mask TypeOptions arith_type: Signed | Unsigned
  simple_bram_vacc37 : Subsystem  AncestorBlock=casper_library_accumulators/simple_bram_vacc  mask(simple_bram_vacc){vec_len=vacc_len, arith_type=Signed, n_bits=32, bin_pt=0}
      mask prompts: vec_len "Vector length:"; arith_type "Output type:"; n_bits "Bit width (output):"; bin_pt "Binary point (output):"
      mask help: This simple vector accumulator is based on a shift register. It outputs its previous accumulated vector after a new_acc pulse is received.
      mask init:
      | simple_bram_vacc_init(gcb, ...
      |     'vec_len', vec_len, ...
      |     'arith_type', arith_type, ...
      |     'n_bits', n_bits, ...
      |     'bin_pt', bin_pt);
      mask TypeOptions arith_type: Signed | Unsigned
  dout : Outport
  vld : Outport  Port=2
  wires:
  din/1 -> c_to_ri/1
  simple_bram_vacc36/2(valid) -> vld/1
  simple_bram_vacc37/1(dout) -> ri_to_c/2
  simple_bram_vacc36/1(dout) -> ri_to_c/1
  c_to_ri/2 -> simple_bram_vacc37/2(din)
  new_acc/1 -> simple_bram_vacc36/1(new_acc), simple_bram_vacc37/1(new_acc)
  c_to_ri/1 -> simple_bram_vacc36/2(din)
  simple_bram_vacc37/2(valid) -> ?
  ri_to_c/1 -> dout/1
